simulink model "QPSK_coarse_synch"  (R2014b)
settings: Solver=ode45  StartTime=0.0  StopTime=5  RelTol=1e-3
PreLoadFcn:
  | %%%%%%%%%%%%%%%%%%%%%%%%%%%%%%%%%%%%%%%%%%%%%%%%%%%%%%%%%%%%%%%%%%%%%%%%%%%
  | % check to see if Simulink library folder is missing from the MATLAB path %
  | %%%%%%%%%%%%%%%%%%%%%%%%%%%%%%%%%%%%%%%%%%%%%%%%%%%%%%%%%%%%%%%%%%%%%%%%%%%
  | if isempty(strfind(path, 'rtlsdr_book_library'))
  | 
  |     % create error window
  |     fig_error = figure(...
  |         'Name', 'Error: RTL-SDR Book Library',...
  |         'Toolbar','none',...
  |         'MenuBar','none',...
  |         'NumberTitle','off',...
  |         'Resize','off',...
  |         'WindowStyle','modal');
  |     fig_error.Position(3) = 600;
  |     fig_error.Position(4) = 150;
  |     fig_axes = axes(...
  |         'Parent',fig_error,...
  |         'Position',[0,0,1,1],...
  |         'visible','off');
  |     % error message
  |     t_title = text(.05,.8,...
  |         'MISSING DIRECTORIES',...
  |         'FontSize',11.5);
  |     t_body = text(.075,.6,...
  |         [{'Simulink cannot find the  \it{<root>}\rm / \it{rtlsdr\_book\_library}\rm  folder in the \it{MATLAB Path}\rm.'},...
  |         {'Please set the MATLAB path following the instructions given in Exercise 2.4.'}],...
  |         'FontSize',10.5);
  |     % buttons
  |     btn_path = uicontrol(...
  |         'Parent',fig_error,...
  |         'String','Set Path Now',...
  |         'FontSize',10,...
  |         'Callback', 'pathtool; close(fig_error);',...
  |         'Position', [fig_error.Position(3)/2-210, 30, 200, 30]);
  |     btn_abort = uicontrol(...
  |         'Parent',fig_error,...
  |         'String','No thanks',...
  |         'FontSize',10,...
  |         'Callback', 'close(fig_error); abort=1;',...
  |         'Position', [fig_error.Position(3)/2+10, 30, 200, 30]);
  | 
  |     % pause to allow user to interact with error box
  |     uiwait(fig_error);
  | 
  |     % abort simulation
  |     try
  |         if abort==1
  |             set_param(gcs, 'SimulationCommand', 'stop');
  |         end
  |     end
  | 
  |     % if user has set path, allow diagram to be updated
  |     if ~exist('abort','var')
  |         % create error window
  |         fig_update = figure(...
  |             'Name', 'Update Diagram',...
  |             'Toolbar','none',...
  |             'MenuBar','none',...
  |             'NumberTitle','off',...
  |             'Resize','off');
  |         fig_update.Position(3) = 400;
  |         fig_update.Position(4) = 120;
  |         fig_axes = axes(...
  |             'Parent',fig_update,...
  |             'Position',[0,0,1,1],...
  |             'visible','off');
  |         % instruction message
  |         t_body = text(.075,.7,...
  |             'Once you have set the path, update the block diagram',...
  |             'FontSize',10.5);
  |         % button
  |         btn_update = uicontrol(...
  |             'Parent',fig_update,...
  |             'String','Update Block Diagram',...
  |             'FontSize',10,...
  |             'Callback', 'set_param(gcs,''SimulationCommand'',''update''); close(gcf)',...
  |             'Position', [fig_update.Position(3)/2-100, 30, 200, 30]);
  |     end
  | 
  |     % clear error components
  |     clear('fig_error','fig_update','fig_axes','t_title','t_body','btn_path','btn_abort','btn_update','abort');
  | 
  | end
  | %%%%%%%%%%%%%%%%%%%%%%%%%%%%%%%%%%%%%%%%%%%%%%%%%%%%%%%%%%%%%%%%%%%%%%%%%%%
  | 
  | 
  | % ---------------- system parameters ------------------
  | 
  | fs_Tx = 240e3;                           % sampling rate used in the transmitter
  | samp = 50000 - 1;                      % stop time (number of samples in the simulation - 1)
  | fc = 60e3;                                  % carrier frequency (IF modulated)
  | Rdata = 2e3;                               % slow data rate chosen for real time demonstration
  | Rsymbol = Rdata/2;                     % QPSK, so 2 samples per symbol
  | fs_Rx = 240e3;                            % sampling rate in the receiver
  | RxDec1 = 5;                                 % decimation at input of Receiver
  | RxDec2 = 6;                                % decimation prior to Coarse Synch
  | RxInt = 3;                                   % interpolation prior to timing and freq synch (output of coarse)
  | OSR = (fs_Rx*RxInt/(RxDec1*RxDec2))/Rsymbol;     % oversampling ratio used in timing and frequency synch
  | 
  | % ---------------- synch loop design ------------------
  | 
  | d = 0.707;                         % damping ratio (using the same for both loops)
  | 
  | % *** CARRIER synch loop *** (note this operates at symbol rate)
  | 
  | T = 1/Rsymbol;                  % sample period
  | Kp = 1;                              % phase detector S-curve is linear
  | Bn = 0.04*Rsymbol;           % bandwidth in Hz
  | Ko = 1;                              % gain of NCO
  | 
  | % calculate the loop filter coefficients for the carrier synch loop
  | K1 = (4*d*Bn*T)/(Ko*Kp*(d+1/(4*d)));
  | K2 = (4*(Bn*T)^2)/(Ko*Kp*(d+1/4*d)^2);
  | 
  | 
  | % *** SYMBOL TIMING synch loop ***
  | 
  | Ts = 1/Rsymbol;                 % symbol period
  | Ks = 3.24;                            % phase detector coefficient
  | BnS = 0.04*Rsymbol;         % bandwidth in Hz
  | Kn   = 1;                            % gain of numerically controlled clock
  | 
  | % calculate loop filter coefficients
  | Ka = (4*d*BnS*Ts)/(Kn*Ks*(d+1/(4*d)));
  | Kb = (4*(BnS*Ts)^2)/(Kn*Ks*(d+1/4*d)^2);
  | 
  | %------------ design of multirate filter objects ----------
  | 
  | Hd1 = mfilt.firdecim(RxDec1);            % first stage decimation
  | Hd2 = mfilt.firdecim(RxDec2);            % second stage decimation
  | 
  | hdC = mfilt.cascade(Hd1,Hd2);           % cascade formed from two decimation stages
  | 
  | %h = fvtool(hdC,'Fs',fs_Rx)                   % show the cascaded decimation filter response
  | 
  | Hi = mfilt.firinterp(RxInt);                   % interpolation
StopFcn:
  | figure(101)
  | subplot(2,1,1)
  | plot(fft_bin.time,squeeze(fft_bin.signals.values),'b');
  | xlabel('Time');
  | ylabel('FFT Bin Number');
  | subplot(2,1,2)
  | plot(freq_offset.time,squeeze(freq_offset.signals.values),'r');
  | xlabel('Time');
  | ylabel('Measured Frequency Offset');
  | 
  | setStandardFigSize(101);
  | set(101,'Name','Peak FFT Bin and Frequency Offset Estimate','NumberTitle','off');
undefined symbols (not defined in the file or in its folder): gcbh, rcfiltgaincompat, startfcn_spectrum_analyzer
libraries: dsparch4 x2, commfilt2 x2, commrandsrc2 x1, commdigbbndpm3 x1, dspspect3 x1, dspstat3 x1, commrflib2 x1, dspmlti4 x1, rtlsdr_book_library x1
CloseFcn:
  | closefcn_model;
Description:
  | Software, Simulation Examples and Design Exercises Licence Agreement
  | 
  | This license agreement refers to the simulation examples, design exercises and files,
  | and associated software MATLAB and Simulink resources that accompany the book:
  | 
  |      Title: Software Defined Radio using MATLAB & Simulink and the RTL-SDR
  |      Published by Strathclyde Academic Media, 2015
  |      Authored by Robert W. Stewart, Kenneth W. Barlee, Dale S.W. Atkinson,
  |      and Louise H. Crockett
  | 
  | and made available as a download from, www.desktopSDR.com or variously acquired
  | by other means such as via USB storage, cloud storage, disk or any other electronic
  | or optical or magnetic storage mechanism. These files and associated software may
  | be used subject to the terms of agreement of the conditions below:
  | 
  |     Copyright © 2015 Robert W. Stewart, Kenneth W. Barlee, Dale S.W. Atkinson,
  |     and Louise H. Crockett
  |     All rights reserved.
  | 
  | Redistribution and use in source and binary forms, with or without modification, are
  | permitted provided that the following conditions are met:
  | 
  |    1.  Redistributions of source code must retain the above copyright notice, this list of
  |         conditions and the following disclaimer.
  | 
  |    2.  Redistributions in binary form must reproduce the above copyright notice, this
  |         list of conditions and the following disclaimer in the documentation and/or other
  |         materials provided with the distribution.
  | 
  |    3.  Neither the name of the copyright holder nor the names of its contributors may
  |         be used to endorse or promote products derived from this software without
  |         specific prior written permission.
  | 
  |    4.  In all cases, the software is, and all modifications and derivatives of the
  |         software shall be, licensed to you solely for use in conjunction with The
  |         MathWorks, Inc. products and service offerings.
  | 
  | THIS SOFTWARE IS PROVIDED BY THE COPYRIGHT HOLDERS AND CONTRIBUTORS
  | "AS IS" AND ANY EXPRESS OR IMPLIED WARRANTIES, INCLUDING, BUT NOT LIMITED
  | TO, THE IMPLIED WARRANTIES OF MERCHANTABILITY AND FITNESS FOR A
  | PARTICULAR PURPOSE ARE DISCLAIMED. IN NO EVENT SHALL THE COPYRIGHT
  | HOLDER OR CONTRIBUTORS BE LIABLE FOR ANY DIRECT, INDIRECT, INCIDENTAL,
  | SPECIAL, EXEMPLARY, OR CONSEQUENTIAL DAMAGES (INCLUDING, BUT NOT
  | LIMITED TO, PROCUREMENT OF SUBSTITUTE GOODS OR SERVICES; LOSS OF USE,
  | DATA, OR PROFITS; OR BUSINESS INTERRUPTION) HOWEVER CAUSED AND ON ANY
  | THEORY OF LIABILITY, WHETHER IN CONTRACT, STRICT LIABILITY, OR TORT
  | (INCLUDING NEGLIGENCE OR OTHERWISE) ARISING IN ANY WAY OUT OF THE USE
  | OF THIS SOFTWARE, EVEN IF ADVISED OF THE POSSIBILITY OF SUCH DAMAGE.
  | 
  | 
  | Audio Tracks used in Simulations Examples and Design Exercises
  | 
  | The music and vocal files used within the Examples files and software within the book
  | were variously written, arranged, performed, recorded and produced by Garrey Rice,
  | Adam Struth, Jamie Struth, Iain Thistlethwaite and also Marshall Craigmyle who
  | collectively, and individually where appropriate, assert and retain all of their copyright,
  | performance and artistic rights. Permission to use and reproduce this music is
  | granted for all purposes associated with MATLAB and Simulink software and the
  | simulation examples and design exercises files that accompany this book. Requests to
  | use the music for any other purpose should be directed to: info@desktopSDR.com.
  | For information on music track names, full credits, and links to the musicians please
  | refer to www.desktopSDR.com/more/audio.
settings Model: Creator=desktopSDR Team  LastModifiedBy=desktopSDR Team
settings DataIOCC: LimitDataPoints=off  SaveOutput=off  SignalLogging=off  SaveTime=off
settings DebuggingCC: UnderspecifiedInitializationDetection=Classic  MergeDetectMultiDrivingBlocksExec=none

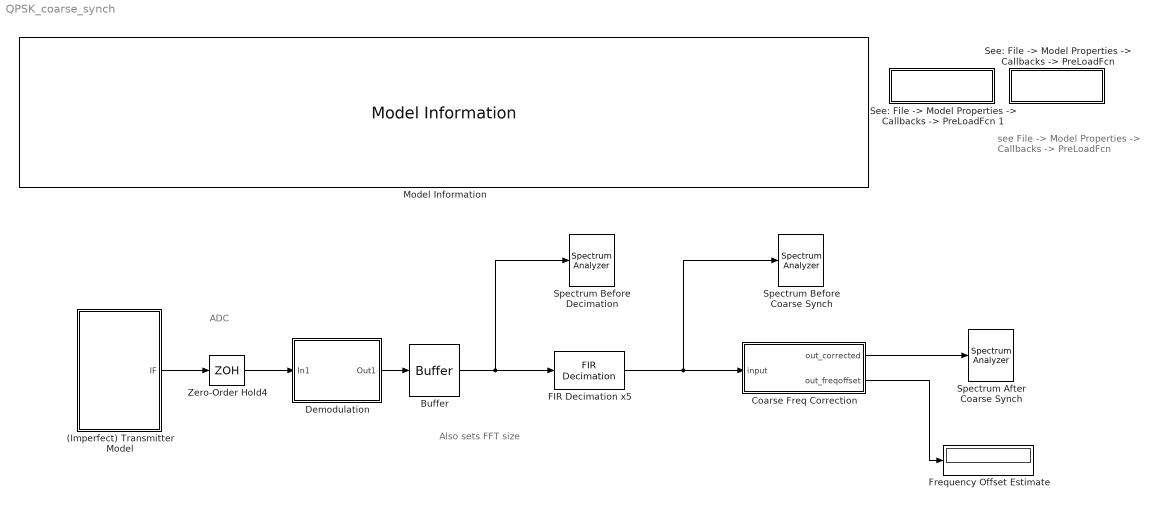
== system QPSK_coarse_synch ==
  note: Also sets
      | FFT size
  note: see File -> Model Properties
      | -> Callbacks -> PreLoadFcn
  note: ADC
  (Imperfect) Transmitter Model : Subsystem  mask(Model of a QPSK Transmitter with Timing and Frequency Offsets){T_error=25, F_error=400}
      mask prompts: T_error "Timing Error (ppm)"; F_error "Frequency Error (Hz)"
      mask help:
      | Enter the timing and frequency offsets that apply to the received signal.
      |
      | Both of these can be negative or positive values. Negative means that the timing / frequency of the transmitter is lower than expected.
      mask init:
      | T_Offset = 1+(T_error/1e6);
      | F_Offset = F_error;
  Buffer : Buffer  N=4096  TreatMby1Signals=One channel
  Coarse Freq Correction : Subsystem
  Demodulation : Subsystem
  FIR Decimation x5 : dspmlti4/FIR Decimation  h=fir1(35,1/5)  D=5  filtStruct=Direct form  framing=Allow multirate processing  inputOffset=0  outputBufInitCond=0  InputProcessing=Columns as channels (frame based)  firstCoeffDataTypeStr=Inherit: Same word length as input  firstCoeffLastDataTypeStr=Inherit: Same word length as input  firstCoeffMin=[]  firstCoeffMax=[]  outputDataTypeStr=Inherit: Same as accumulator  outputLastDataTypeStr=Inherit: Same as accumulator  outputMin=[]  outputMax=[]  roundingMode=Floor  overflowMode=off  FilterSource=Filter object  FilterObject=Hd1
      settings: allowOverrides=off
  Frequency Offset Estimate : Display
  Model Information : rtlsdr_book_library/Additional Tools/Model Information/Model Information
  "See: File -> Model Properties -> Callbacks -> PreLoadFcn " : Subsystem
      mask Display:
      | fs_Rx = evalin('base', 'fs_Rx');
      | fprintf(['fs_Rx = ',num2str(fs_Rx/1e3),' kHz']);
  "See: File -> Model Properties -> Callbacks -> PreLoadFcn 1" : Subsystem
      mask Display:
      | Rsymbol = evalin('base', 'Rsymbol');
      | fprintf(['Rsymbol = ',num2str(Rsymbol/1e3),' ksps']);
  Spectrum After Coarse Synch : SpectrumAnalyzer  StartFcn=startfcn_spectrum_analyzer;
  Spectrum Before Coarse Synch : SpectrumAnalyzer  StartFcn=startfcn_spectrum_analyzer;
  Spectrum Before Decimation : SpectrumAnalyzer  StartFcn=startfcn_spectrum_analyzer;
  Zero-Order Hold4 : ZeroOrderHold  SampleTime=1/fs_Rx
  wires:
  Coarse Freq Correction/2(out_freqoffset) -> Frequency Offset Estimate/1
  Coarse Freq Correction/1(out_corrected) -> Spectrum After Coarse Synch/1
  Buffer/1 -> FIR Decimation x5/1, Spectrum Before Decimation/1
  (Imperfect) Transmitter Model/1(IF) -> Zero-Order Hold4/1
  Zero-Order Hold4/1 -> Demodulation/1(In1)
  Demodulation/1(Out1) -> Buffer/1
  FIR Decimation x5/1 -> Coarse Freq Correction/1(input), Spectrum Before Coarse Synch/1

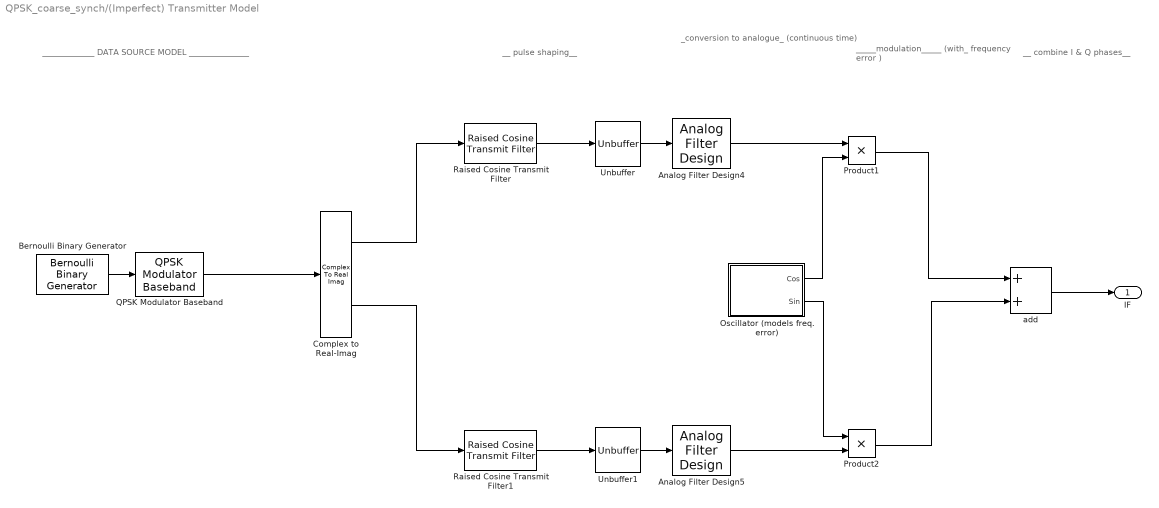
== system QPSK_coarse_synch/(Imperfect) Transmitter Model ==
  note: _____________ DATA SOURCE MODEL _______________
  note: _conversion to analogue_
      | (continuous time)
  note: __ pulse shaping__
  note: _____modulation_____
      | (with_ frequency error )
  note: __ combine I & Q phases__
  Analog Filter Design4 : dsparch4/Analog Filter Design  method=Butterworth  filttype=Lowpass  N=8  Wlo=2*pi*Rsymbol*T_Offset  Whi=80  Rp=2  Rs=40
  Analog Filter Design5 : dsparch4/Analog Filter Design  method=Butterworth  filttype=Lowpass  N=8  Wlo=2*pi*Rsymbol*T_Offset  Whi=80  Rp=2  Rs=40
  Bernoulli Binary Generator : commrandsrc2/Bernoulli Binary Generator  P=0.5  seed=61  Ts=1/(T_Offset*Rdata)  frameBased=on  sampPerFrame=2  orient=off  outDataType=double
  Complex to Real-Imag : ComplexToRealImag
  Oscillator (models freq. error) : Subsystem
  Product1 : Product
  Product2 : Product
  QPSK Modulator Baseband : commdigbbndpm3/QPSK Modulator Baseband  InType=Bit  Enc=Gray  Ph=pi/4  outDtype=double  outWordLen=16  outUDDataType=sfix(16)  outFracLenMode=Best precision  outFracLen=15
  Raised Cosine Transmit Filter : commfilt2/Raised Cosine Transmit Filter  filtType=Square root  filtSpan=12  currentFiltSpan=2*((12)/2)  D=(12)/2  R=0.5  sampMode=Mute  saveAsFlag=0  N=fs_Tx/Rsymbol  framing=Allow multirate processing  InputProcessing=Columns as channels (frame based)  checkGain=Normalized  filterGain=rcfiltgaincompat(gcbh)  checkCoeff=off  variableName=rcTxFilt  launchFVT=on  roundingMode=Floor  overflowMode=off
  Raised Cosine Transmit Filter1 : commfilt2/Raised Cosine Transmit Filter  filtType=Square root  filtSpan=12  currentFiltSpan=2*((12)/2)  D=(12)/2  R=0.5  sampMode=Mute  saveAsFlag=0  N=fs_Tx/Rsymbol  framing=Allow multirate processing  InputProcessing=Columns as channels (frame based)  checkGain=Normalized  filterGain=rcfiltgaincompat(gcbh)  checkCoeff=off  variableName=rcTxFilt1  launchFVT=on  roundingMode=Floor  overflowMode=off
  Unbuffer : Unbuffer  SampleBasedProcessing=Same as frame based
  Unbuffer1 : Unbuffer  SampleBasedProcessing=Same as frame based
  add : Sum
  IF : Outport
  wires:
  Raised Cosine Transmit Filter1/1 -> Unbuffer1/1
  Complex to Real-Imag/2 -> Raised Cosine Transmit Filter1/1
  Complex to Real-Imag/1 -> Raised Cosine Transmit Filter/1
  Bernoulli Binary Generator/1 -> QPSK Modulator Baseband/1
  Raised Cosine Transmit Filter/1 -> Unbuffer/1
  Product1/1 -> add/1
  Analog Filter Design4/1 -> Product1/1
  Analog Filter Design5/1 -> Product2/2
  Product2/1 -> add/2
  add/1 -> IF/1
  Oscillator (models freq. error)/1(Cos) -> Product1/2
  Oscillator (models freq. error)/2(Sin) -> Product2/1
  QPSK Modulator Baseband/1 -> Complex to Real-Imag/1
  Unbuffer/1 -> Analog Filter Design4/1
  Unbuffer1/1 -> Analog Filter Design5/1

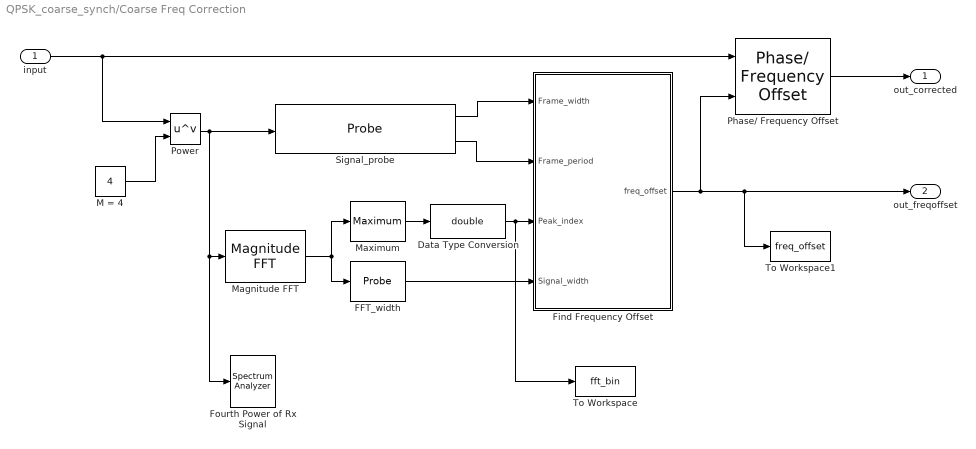
== system QPSK_coarse_synch/Coarse Freq Correction ==
  input : Inport
  Data Type Conversion : DataTypeConversion  OutDataTypeStr=double
  FFT_width : Probe  ProbeSampleTime=off  ProbeComplexSignal=off  ProbeSampleTimeDataType=single
  Find Frequency Offset : MATLAB Function  TreatAsAtomicUnit=on
  Fourth Power of Rx Signal : SpectrumAnalyzer  StartFcn=startfcn_spectrum_analyzer;
  M = 4 : Constant  Value=4  OutDataTypeStr=double
  Magnitude FFT : dspspect3/Magnitude FFT  mag_or_magsq=Magnitude squared  FFTImplementation=Auto  fftLenInherit=on  fftsize=1024  WrapInput=on
  Maximum : dspstat3/Maximum  fcn=Index  reset=None  InputProcessing=Columns as channels (frame based)  indexBase=One  operateOver=Each column  Dimension=1  colComp=on  operation=maximum  roiEnable=off  roiType=Rectangles  roiPortion=Entire ROI  roiOutput=Individual statistics for each ROI  roiFlag=off  accumDataTypeStr=Inherit: Same as product output  accumLastDataTypeStr=Inherit: Same as product output  roundingMode=Floor  overflowMode=off
  Phase/ Frequency Offset : commrflib2/Phase// Frequency Offset  phaseOffset=0  freqPort=on  freqOffset=0
  Power : Math  Operator=pow  OutputSignalType=complex  SaturateOnIntegerOverflow=on
  Signal_probe : Probe  ProbeComplexSignal=off
  To Workspace : ToWorkspace  VariableName=fft_bin  SaveFormat=Structure With Time  SampleTime=-1
  To Workspace1 : ToWorkspace  VariableName=freq_offset  SaveFormat=Structure With Time  SampleTime=-1
  out_corrected : Outport
  out_freqoffset : Outport  Port=2
  wires:
  Power/1 -> Signal_probe/1, Fourth Power of Rx Signal/1, Magnitude FFT/1
  Find Frequency Offset/1(freq_offset) -> Phase/ Frequency Offset/2, To Workspace1/1, out_freqoffset/1
  Signal_probe/2 -> Find Frequency Offset/2(Frame_period)
  FFT_width/1 -> Find Frequency Offset/4(Signal_width)
  M = 4/1 -> Power/2
  Signal_probe/1 -> Find Frequency Offset/1(Frame_width)
  Magnitude FFT/1 -> Maximum/1, FFT_width/1
  input/1 -> Power/1, Phase/ Frequency Offset/1
  Phase/ Frequency Offset/1 -> out_corrected/1
  Maximum/1 -> Data Type Conversion/1
  Data Type Conversion/1 -> To Workspace/1, Find Frequency Offset/3(Peak_index)

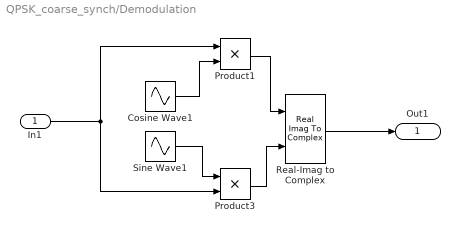
== system QPSK_coarse_synch/Demodulation ==
  In1 : Inport
  Cosine Wave1 : Sin  Amplitude=sqrt(2)  Frequency=fc*2*pi  Phase=pi/2  SampleTime=1/fs_Rx
  Product1 : Product
  Product3 : Product
  Real-Imag to Complex : RealImagToComplex
  Sine Wave1 : Sin  Amplitude=sqrt(2)  Frequency=fc*2*pi  SampleTime=1/fs_Rx
  Out1 : Outport
  wires:
  Product1/1 -> Real-Imag to Complex/1
  Real-Imag to Complex/1 -> Out1/1
  Product3/1 -> Real-Imag to Complex/2
  In1/1 -> Product1/1, Product3/2
  Sine Wave1/1 -> Product3/1
  Cosine Wave1/1 -> Product1/2

== system QPSK_coarse_synch/See: File -> Model Properties -> Callbacks -> PreLoadFcn  ==

== system QPSK_coarse_synch/See: File -> Model Properties -> Callbacks -> PreLoadFcn 1 ==

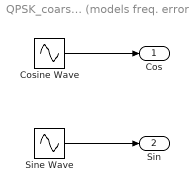
== system QPSK_coarse_synch/(Imperfect) Transmitter Model/Oscillator (models freq. error) ==
  Cosine Wave : Sin  Frequency=2*pi*(fc+F_Offset)  Phase=pi/2  SampleTime=0
  Sine Wave : Sin  Frequency=2*pi*(fc+F_Offset)  SampleTime=0
  Cos : Outport
  Sin : Outport  Port=2
  wires:
  Sine Wave/1 -> Sin/1
  Cosine Wave/1 -> Cos/1

== matlab function QPSK_coarse_synch/Coarse Freq Correction/Find Frequency Offset ==
  data: Frame_width input; freq_offset output; Frame_period input; Peak_index input; Signal_width input
%% Frequency offset calculation
% The code in this function takes the inputs, and uses them to calculate 
% the frequency offset required to synchronise the input signal to baseband. 
%-------------------------------------------------------------------------%
function freq_offset = fcn(Frame_width,Frame_period,Peak_index,Signal_width)
% Logic to compute required index offset value
if Peak_index > Signal_width/2
    offset = (Signal_width+1)-Peak_index;
else
    offset = 1-Peak_index;
end

% Convert offset to a frequency shift value.
% calculate sample time
Ts = Frame_period(1)/Frame_width;
% calculate frequency resolution of the FFT signal
freq_resolution = 1/(Ts*Signal_width);
% compute frequency offset using this value
freq_offset = offset * freq_resolution/4;
